simulink model "TriggeredIntegrator"  (R2020b)
settings: Solver=VariableStepAuto  StartTime=0.0  StopTime=10.0  RelTol=1e-3
settings Model: Creator=pgoldschmid  LastModifiedBy=pgoldschmid

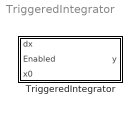
== system TriggeredIntegrator ==
  TriggeredIntegrator : Subsystem  TreatAsAtomicUnit=on

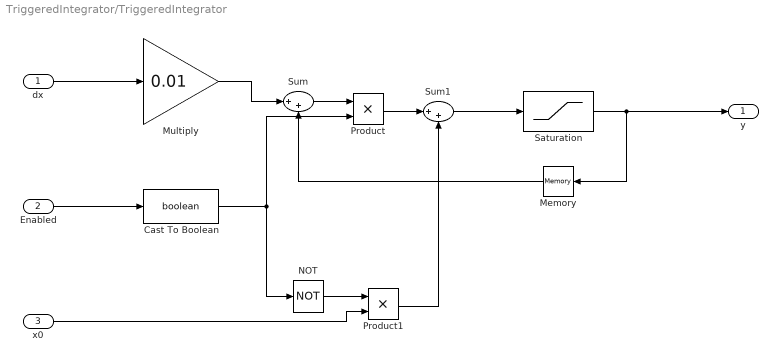
== system TriggeredIntegrator/TriggeredIntegrator ==
  dx : Inport
  Enabled : Inport  Port=2
  x0 : Inport  Port=3
  Cast To Boolean : DataTypeConversion  OutDataTypeStr=boolean
  Memory : Memory
  Multiply : Gain  Gain=0.01  OutDataTypeStr=Inherit: Same as input
  NOT : Logic  Operator=NOT  IconShape=distinctive  AllPortsSameDT=off  OutDataTypeStr=boolean
  Product : Product
  Product1 : Product
  Saturation : Saturate  UpperLimit=50  LowerLimit=-2
  Sum : Sum  Inputs=|++
  Sum1 : Sum  Inputs=|++
  y : Outport
  wires:
  Multiply/1 -> Sum/1
  Memory/1 -> Sum/2
  Saturation/1 -> y/1, Memory/1
  Sum/1 -> Product/1
  dx/1 -> Multiply/1
  Enabled/1 -> Cast To Boolean/1
  Cast To Boolean/1 -> Product/2, NOT/1
  Product1/1 -> Sum1/2
  NOT/1 -> Product1/1
  Product/1 -> Sum1/1
  Sum1/1 -> Saturation/1
  x0/1 -> Product1/2
